simulink model "Despegue_model"  (R2015b)
settings: Solver=ode45  StartTime=0  StopTime=1000  FixedStep=0.001  RelTol=1e-3
libraries: simulink_extras x4, aerolibtransform2 x2, aerolibutil x2, simulink x1, aerolibobsolete x1, aerolibasang x1
settings Model: Creator=David  LastModifiedBy=Juan
settings SolverCC: InitialStep=AUTO
settings DataIOCC: SaveCompleteFinalSimState=on  SaveFormat=Array  SaveState=on  ReturnWorkspaceOutputsName=simout
settings DebuggingCC: AlgebraicLoopMsg=none  UnderspecifiedInitializationDetection=Classic  MergeDetectMultiDrivingBlocksExec=none  StateNameClashWarn=warning
settings HardwareCC: ProdBitPerPointer=32  ProdLargestAtomicFloat=None  ProdIntDivRoundTo=Undefined  ProdEndianess=Unspecified  ProdWordSize=32  ProdHWDeviceType=32-bit Generic
settings GRTTargetCC: GeneratePreprocessorConditionals=Disable all
settings ConfigComp: CovModelRefEnable=Off

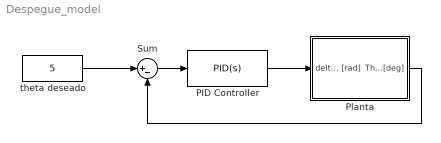
== system Despegue_model ==
  PID Controller : simulink/Continuous/PID Controller  Controller=PID  TimeDomain=Continuous-time  SampleTime=-1  IntegratorMethod=Forward Euler  FilterMethod=Forward Euler  Form=Parallel  UseFilter=on  ControllerParametersSource=internal  P=-0.450238898063441  I=-0.00789924414267895  D=0.0642858198815756  N=2  InitialConditionSource=internal  InitialConditionForIntegrator=0  InitialConditionForFilter=0  ExternalReset=none  LimitOutput=on  UpperSaturationLimit=0.062  LowerSaturationLimit=-0.062  LinearizeAsGain=on  AntiWindupMode=none  Kb=1  TrackingMode=off  Kt=1  PParamMin=[]  PParamMax=[]  IParamMin=[]  IParamMax=[]  DParamMin=[]  DParamMax=[]  NParamMin=[]  NParamMax=[]  KbParamMin=[]  KbParamMax=[]  KtParamMin=[]  KtParamMax=[]  POutMin=[]  POutMax=[]  IOutMin=[]  IOutMax=[]  DOutMin=[]  DOutMax=[]  NOutMin=[]  NOutMax=[]  KbOutMin=[]  KbOutMax=[]  KtOutMin=[]  KtOutMax=[]  IntegratorOutMin=[]  IntegratorOutMax=[]  FilterOutMin=[]  FilterOutMax=[]  SumOutMin=[]  SumOutMax=[]  SumI1OutMin=[]  SumI1OutMax=[]  SumI2OutMin=[]  SumI2OutMax=[]  SumI3OutMin=[]  SumI3OutMax=[]  SumDOutMin=[]  SumDOutMax=[]  SaturationOutMin=[]  SaturationOutMax=[]  IntegratorContinuousStateAttributes=''  IntegratorStateMustResolveToSignalObject=off  IntegratorRTWStateStorageClass=Auto  FilterContinuousStateAttributes=''  FilterStateMustResolveToSignalObject=off  FilterRTWStateStorageClass=Auto  DifferentiatorICPrevScaledInput=0  DifferentiatorOutMin=[]  DifferentiatorOutMax=[]
  Planta : Subsystem
  Sum : Sum  Inputs=|+-
  theta deseado : Constant  Value=5
  wires:
  Planta/1(Theta[deg]) -> Sum/2
  Sum/1 -> PID Controller/1
  theta deseado/1 -> Sum/1
  PID Controller/1 -> Planta/1(delta [rad])

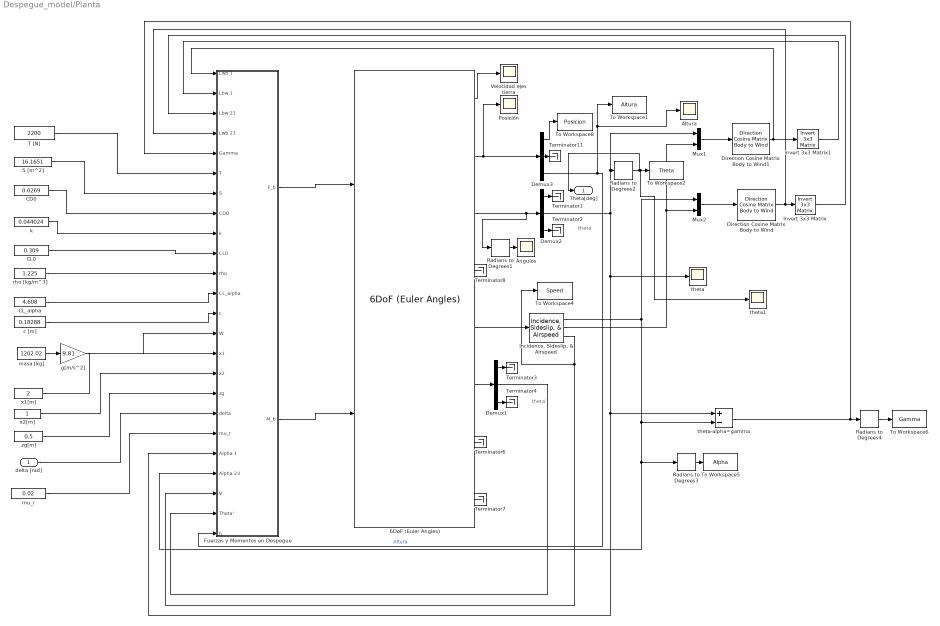
== system Despegue_model/Planta ==
  note: theta'
  note: theta
  delta [rad] : Inport
  6DoF (Euler Angles) : aerolibobsolete/6DoF (Euler Angles)  units=Metric (MKS)  mtype=Fixed  rep=Euler Angles  xme_0=[0 0 0]  Vm_0=[0.01 0 0]  eul_0=[0 0.035 0]  pm_0=[0 0 0]  mass_0=Mass  mass_e=0.5  mass_f=2.0  inertia=Inertia  inertia_e=eye(3)  inertia_f=2*eye(3)  k_quat=1.0
  Altura : Scope
  CD0 : Constant  Value=0.0269
  CL0 : Constant  Value=0.309
  "CL_alpha " : Constant  Value=4.608
  Demux1 : Demux  Outputs=3
  Demux2 : Demux  Outputs=3
  Demux3 : Demux  Outputs=3
  Direction Cosine Matrix Body to Wind : aerolibtransform2/Direction Cosine Matrix Body to Wind
  Direction Cosine Matrix Body to Wind1 : aerolibtransform2/Direction Cosine Matrix Body to Wind
  Fuerzas y Momentos en Despegue : Subsystem
  "Incidence, Sideslip, & Airspeed" : aerolibasang/Incidence, Sideslip, & Airspeed
  Invert 3x3 Matrix : aerolibutil/Invert  3x3 Matrix
  Invert 3x3 Matrix1 : aerolibutil/Invert  3x3 Matrix
  Mux1 : Mux  Inputs=2
  Mux2 : Mux  Inputs=2
  Posición : Scope
  Radians to Degrees{1..4} (4 alike) : simulink_extras/Transformations/Radians to Degrees
  S [m^2] : Constant  Value=16.1651
  T [N] : Constant  Value=2200
  Terminator{1..4,6..8,11} (8 alike) : Terminator
  To Workspace1 : ToWorkspace  VariableName=Altura  SampleTime=-1
  To Workspace2 : ToWorkspace  VariableName=Theta  SampleTime=-1
  To Workspace4 : ToWorkspace  VariableName=Speed  SampleTime=-1
  To Workspace5 : ToWorkspace  VariableName=Alpha  SampleTime=-1
  To Workspace6 : ToWorkspace  VariableName=Gamma  SampleTime=-1
  To Workspace8 : ToWorkspace  VariableName=Posicion  SampleTime=-1
  "Velocidad ejes tierra " : Scope
  c [m] : Constant  Value=0.18288
  g[m/s^2] : Gain  Gain=9.81
  k : Constant  Value=0.044024
  "masa [kg] " : Constant  Value=1202.02
  "mu_r " : Constant  Value=0.02
  rho [kg/m^3] : Constant  Value=1.225
  theta : Scope
  theta-alpha=gamma : Sum  Inputs=+-
  theta1 : Scope
  x1[m] : Constant  Value=2
  x2[m] : Constant
  zg[m] : Constant  Value=0.5
  Ángulos : Scope
  Theta[deg] : Outport
  wires:
  6DoF (Euler Angles)/1 -> "Velocidad ejes tierra "/1
  6DoF (Euler Angles)/6 -> Demux1/1
  6DoF (Euler Angles)/7 -> Terminator6/1
  6DoF (Euler Angles)/8 -> Terminator7/1
  Radians to Degrees4/1 -> To Workspace6/1
  T [N]/1 -> Fuerzas y Momentos en Despegue/6(T)
  "Incidence, Sideslip, & Airspeed"/3 -> Fuerzas y Momentos en Despegue/22(V), To Workspace4/1
  Demux2/3 -> Terminator2/1
  Invert 3x3 Matrix1/1 -> Fuerzas y Momentos en Despegue/2(Lbw 1)
  Demux1/1 -> Terminator3/1
  Demux3/2 -> Terminator11/1
  Radians to Degrees1/1 -> Ángulos/1
  S [m^2]/1 -> Fuerzas y Momentos en Despegue/7(S)
  CD0/1 -> Fuerzas y Momentos en Despegue/8(CD0)
  Demux3/1 -> To Workspace8/1
  Demux2/2 -> theta/1, Fuerzas y Momentos en Despegue/20(Alpha 1), theta-alpha=gamma/1, Mux1/1, Radians to Degrees2/1
  6DoF (Euler Angles)/2 -> Demux3/1, Posición/1
  "Incidence, Sideslip, & Airspeed"/2 -> Mux2/2, Mux1/2
  "masa [kg] "/1 -> g[m/s^2]/1
  6DoF (Euler Angles)/5 -> "Incidence, Sideslip, & Airspeed"/1
  6DoF (Euler Angles)/4 -> Terminator8/1
  Demux2/1 -> Terminator1/1
  Mux2/1 -> Direction Cosine Matrix Body to Wind/1
  Direction Cosine Matrix Body to Wind1/1 -> Fuerzas y Momentos en Despegue/1(Lwb 1), Invert 3x3 Matrix1/1
  Direction Cosine Matrix Body to Wind/1 -> Fuerzas y Momentos en Despegue/4(Lwb 23), Invert 3x3 Matrix/1
  Radians to Degrees3/1 -> To Workspace5/1
  theta-alpha=gamma/1 -> Fuerzas y Momentos en Despegue/5(Gamma), Radians to Degrees4/1
  k/1 -> Fuerzas y Momentos en Despegue/9(k)
  Invert 3x3 Matrix/1 -> Fuerzas y Momentos en Despegue/3(Lbw 23)
  Mux1/1 -> Direction Cosine Matrix Body to Wind1/1
  Demux3/3 -> Fuerzas y Momentos en Despegue/24(h), To Workspace1/1, Altura/1  "Altura"
  Radians to Degrees2/1 -> theta1/1, To Workspace2/1, Theta[deg]/1
  Demux1/3 -> Terminator4/1
  6DoF (Euler Angles)/3 -> Radians to Degrees1/1, Demux2/1
  zg[m]/1 -> Fuerzas y Momentos en Despegue/17(zg)
  CL0/1 -> Fuerzas y Momentos en Despegue/10(CL0)
  Demux1/2 -> Fuerzas y Momentos en Despegue/23(Theta')
  rho [kg/m^3]/1 -> Fuerzas y Momentos en Despegue/11(rho)
  "CL_alpha "/1 -> Fuerzas y Momentos en Despegue/12(CL_alpha)
  c [m]/1 -> Fuerzas y Momentos en Despegue/13(c)
  Fuerzas y Momentos en Despegue/1(F_b) -> 6DoF (Euler Angles)/1
  g[m/s^2]/1 -> Fuerzas y Momentos en Despegue/14(W)
  x1[m]/1 -> Fuerzas y Momentos en Despegue/15(x1)
  x2[m]/1 -> Fuerzas y Momentos en Despegue/16(x2)
  "mu_r "/1 -> Fuerzas y Momentos en Despegue/19(mu_r)
  Fuerzas y Momentos en Despegue/2(M_b) -> 6DoF (Euler Angles)/2
  delta [rad]/1 -> Fuerzas y Momentos en Despegue/18(delta)
  "Incidence, Sideslip, & Airspeed"/1 -> Mux2/1, Radians to Degrees3/1, Fuerzas y Momentos en Despegue/21(Alpha 23), theta-alpha=gamma/2

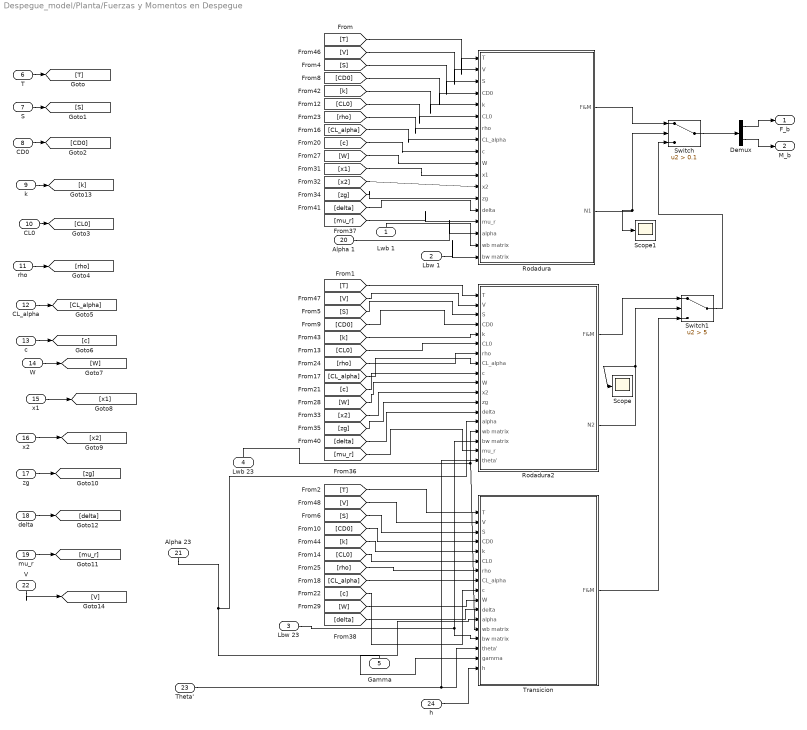
== system Despegue_model/Planta/Fuerzas y Momentos en Despegue ==
  Lwb 1 : Inport
  Lbw 1 : Inport  Port=2
  Lbw 23 : Inport  Port=3
  Lwb 23 : Inport  Port=4
  Gamma : Inport  Port=5
  T : Inport  Port=6
  S : Inport  Port=7
  CD0 : Inport  Port=8
  k : Inport  Port=9
  CL0 : Inport  Port=10
  rho : Inport  Port=11
  CL_alpha : Inport  Port=12
  c : Inport  Port=13
  W : Inport  Port=14
  x1 : Inport  Port=15
  x2 : Inport  Port=16
  zg : Inport  Port=17
  delta : Inport  Port=18
  mu_r : Inport  Port=19
  Alpha 1 : Inport  Port=20
  Alpha 23 : Inport  Port=21
  V : Inport  Port=22
  Theta' : Inport  Port=23
  h : Inport  Port=24
  Demux : Demux  Outputs=2
  Rodadura : Subsystem
  Rodadura2 : Subsystem
  Scope : Scope
  Scope1 : Scope
  Switch : Switch  Criteria=u2 > Threshold  Threshold=0.1
  Switch1 : Switch  Criteria=u2 > Threshold  Threshold=5  ZeroCross=off
  Transicion : Subsystem
  F_b : Outport
  M_b : Outport  Port=2
  wires:
  Alpha 1/1 -> Rodadura/16(alpha)
  Alpha 23/1 -> Transicion/12(alpha), Rodadura2/14(alpha)
  Gamma/1 -> Transicion/16(gamma)
  Lwb 23/1 -> Transicion/13(wb matrix), Rodadura2/15(wb matrix)
  Rodadura/1(F&M) -> Switch/1
  Theta'/1 -> Transicion/15(theta'), Rodadura2/18(theta')
  Switch1/1 -> Switch/3
  Switch/1 -> Demux/1
  Lbw 23/1 -> Transicion/14(bw matrix), Rodadura2/16(bw matrix)
  Rodadura2/1(F&M) -> Switch1/1
  Demux/2 -> M_b/1
  Lbw 1/1 -> Rodadura/18(bw matrix)
  Rodadura2/2("N2 ") -> Scope/1, Switch1/2
  Demux/1 -> F_b/1
  T/1 -> [T]
  [T] -> Rodadura/1(T)
  [T] -> Rodadura2/1(T)
  [T] -> Transicion/1(T)
  S/1 -> [S]
  CD0/1 -> [CD0]
  CL0/1 -> [CL0]
  rho/1 -> [rho]
  CL_alpha/1 -> [CL_alpha]
  c/1 -> [c]
  W/1 -> [W]
  x1/1 -> [x1]
  x2/1 -> [x2]
  zg/1 -> [zg]
  [S] -> Rodadura/3(S)
  [S] -> Rodadura2/3(S)
  [S] -> Transicion/3(S)
  [CD0] -> Rodadura/4(CD0)
  [CD0] -> Rodadura2/4(CD0)
  [CD0] -> Transicion/4(CD0)
  [CL0] -> Rodadura/6(CL0)
  [CL0] -> Rodadura2/6(CL0)
  [CL0] -> Transicion/6(CL0)
  [CL_alpha] -> Rodadura/8(CL_alpha)
  [CL_alpha] -> Rodadura2/8(CL_alpha)
  [CL_alpha] -> Transicion/8(CL_alpha)
  [c] -> Rodadura/9(c)
  [c] -> Rodadura2/9(c)
  [c] -> Transicion/9(c)
  [rho] -> Rodadura/7(rho)
  [rho] -> Rodadura2/7(rho)
  [rho] -> Transicion/7(rho)
  [W] -> Rodadura/10(W)
  [W] -> Rodadura2/10(W)
  [W] -> Transicion/10(W)
  [x1] -> Rodadura/11(x1)
  [x2] -> Rodadura/12(x2)
  [x2] -> Rodadura2/11(x2)
  [zg] -> Rodadura/13(zg)
  [zg] -> Rodadura2/12(zg)
  mu_r/1 -> [mu_r]
  [mu_r] -> Rodadura2/17(mu_r)
  [mu_r] -> Rodadura/15(mu_r)
  delta/1 -> [delta]
  [delta] -> Transicion/11(delta)
  [delta] -> Rodadura2/13(delta)
  [delta] -> Rodadura/14(delta)
  k/1 -> [k]
  [k] -> Rodadura/5(k)
  [k] -> Rodadura2/5(k)
  [k] -> Transicion/5(k)
  V/1 -> [V]
  [V] -> Rodadura/2(V)
  [V] -> Rodadura2/2(V)
  [V] -> Transicion/2(V)
  Lwb 1/1 -> Rodadura/17(wb matrix)
  Transicion/1(F&M) -> Switch1/3
  Rodadura/2("N1 ") -> Switch/2, Scope1/1
  h/1 -> Transicion/17(h)

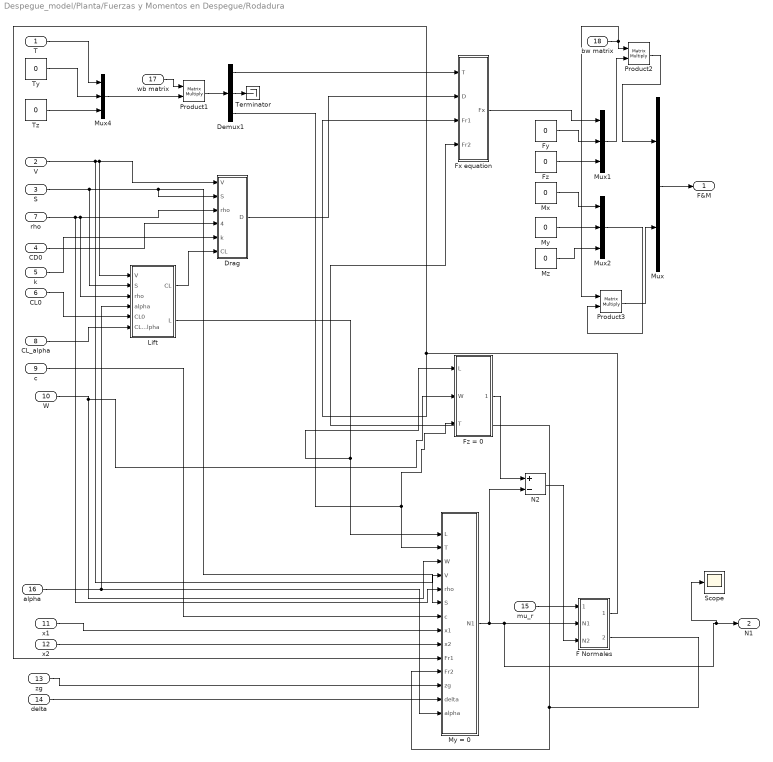
== system Despegue_model/Planta/Fuerzas y Momentos en Despegue/Rodadura ==
  T : Inport
  V : Inport  Port=2
  S : Inport  Port=3
  CD0 : Inport  Port=4
  k : Inport  Port=5
  CL0 : Inport  Port=6
  rho : Inport  Port=7
  CL_alpha : Inport  Port=8
  c : Inport  Port=9
  W : Inport  Port=10
  x1 : Inport  Port=11
  x2 : Inport  Port=12
  zg : Inport  Port=13
  delta : Inport  Port=14
  mu_r : Inport  Port=15
  alpha : Inport  Port=16
  wb matrix : Inport  Port=17
  bw matrix : Inport  Port=18
  Demux1 : Demux  Outputs=3
  Drag : Subsystem
  F Normales : Subsystem
  Fx equation : Subsystem
  Fy : Constant  Value=0
  Fz : Constant  Value=0
  Fz = 0 : Subsystem
  Lift : Subsystem
  Mux : Mux  Inputs=2
  Mux1 : Mux  Inputs=3
  Mux2 : Mux  Inputs=3
  Mux4 : Mux  Inputs=3
  Mx : Constant  Value=0
  My : Constant  Value=0
  My = 0 : Subsystem
  Mz : Constant  Value=0
  N2 : Sum  Inputs=+-
  Product1 : Product  Multiplication=Matrix(*)
  Product2 : Product  Multiplication=Matrix(*)
  Product3 : Product  Multiplication=Matrix(*)
  Scope : Scope
  Terminator : Terminator
  Ty : Constant  Value=0
  Tz : Constant  Value=0
  F&M : Outport
  "N1 " : Outport  Port=2
  wires:
  Mux/1 -> F&M/1
  Fz/1 -> Mux1/3
  Mx/1 -> Mux2/1
  Mz/1 -> Mux2/3
  T/1 -> Mux4/1
  Ty/1 -> Mux4/2
  Tz/1 -> Mux4/3
  Mux4/1 -> Product1/2
  Lift/1(CL) -> Drag/6(CL)
  Lift/2(L) -> My = 0/1(L), Fz = 0/1(L)
  Drag/1(D) -> Fx equation/2(D)
  My = 0/1(N1) -> N2/2, Scope/1, "N1 "/1, F Normales/2(N1)
  Fz = 0/1(N1+N2) -> N2/1
  N2/1 -> F Normales/3(N2)
  F Normales/1("Fr1 ") -> Fx equation/3(Fr1), My = 0/10(Fr1)
  F Normales/2(Fr2) -> My = 0/11(Fr2), Fx equation/4(Fr2)
  Product1/1 -> Demux1/1
  Demux1/1 -> Fx equation/1(T)
  Demux1/2 -> Terminator/1
  Demux1/3 -> My = 0/2(T), Fz = 0/3(T)
  My/1 -> Mux2/2
  Fy/1 -> Mux1/2
  V/1 -> My = 0/4(V), Lift/1(V), Drag/1(V)
  S/1 -> My = 0/6(S), Drag/2(S), Lift/2(S)
  rho/1 -> Lift/3(rho), Drag/3(rho), My = 0/5(rho)
  CD0/1 -> Drag/4(CD0)
  k/1 -> Drag/5(k)
  CL0/1 -> Lift/5(CL0)
  CL_alpha/1 -> Lift/6(CL_alpha)
  c/1 -> My = 0/7(c)
  W/1 -> My = 0/3(W), Fz = 0/2(W)
  x1/1 -> My = 0/8(x1)
  x2/1 -> My = 0/9(x2)
  zg/1 -> My = 0/12(zg)
  delta/1 -> My = 0/13(delta)
  alpha/1 -> Lift/4(alpha), My = 0/14(alpha)
  mu_r/1 -> F Normales/1(mu_r)
  wb matrix/1 -> Product1/1
  Mux1/1 -> Product2/2
  bw matrix/1 -> Product2/1, Product3/1
  Product2/1 -> Mux/1
  Product3/1 -> Mux/2
  Mux2/1 -> Product3/2
  Fx equation/1(Fx) -> Mux1/1

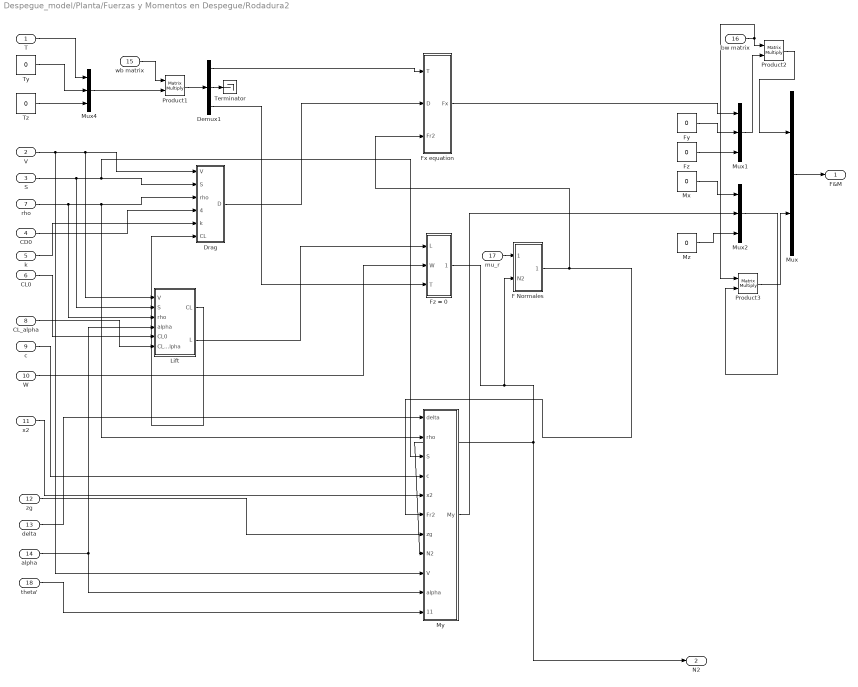
== system Despegue_model/Planta/Fuerzas y Momentos en Despegue/Rodadura2 ==
  T : Inport
  V : Inport  Port=2
  S : Inport  Port=3
  CD0 : Inport  Port=4
  k : Inport  Port=5
  CL0 : Inport  Port=6
  rho : Inport  Port=7
  CL_alpha : Inport  Port=8
  c : Inport  Port=9
  W : Inport  Port=10
  x2 : Inport  Port=11
  zg : Inport  Port=12
  delta : Inport  Port=13
  alpha : Inport  Port=14
  wb matrix : Inport  Port=15
  bw matrix : Inport  Port=16
  mu_r : Inport  Port=17
  theta' : Inport  Port=18
  " My" : Subsystem
  Demux1 : Demux  Outputs=3
  Drag : Subsystem
  F Normales : Subsystem
  Fx equation : Subsystem
  Fy : Constant  Value=0
  Fz : Constant  Value=0
  Fz = 0 : Subsystem
  Lift : Subsystem
  Mux : Mux  Inputs=2
  Mux1 : Mux  Inputs=3
  Mux2 : Mux  Inputs=3
  Mux4 : Mux  Inputs=3
  Mx : Constant  Value=0
  Mz : Constant  Value=0
  Product1 : Product  Multiplication=Matrix(*)
  Product2 : Product  Multiplication=Matrix(*)
  Product3 : Product  Multiplication=Matrix(*)
  Terminator : Terminator
  Ty : Constant  Value=0
  Tz : Constant  Value=0
  F&M : Outport
  "N2 " : Outport  Port=2
  wires:
  Mux/1 -> F&M/1
  Fz/1 -> Mux1/3
  Mx/1 -> Mux2/1
  Mz/1 -> Mux2/3
  T/1 -> Mux4/1
  Ty/1 -> Mux4/2
  Tz/1 -> Mux4/3
  Mux4/1 -> Product1/2
  Lift/1(CL) -> Drag/6(CL)
  Drag/1(D) -> Fx equation/2(D)
  Product1/1 -> Demux1/1
  Demux1/1 -> Fx equation/1(T)
  Demux1/2 -> Terminator/1
  " My"/1(My) -> Mux2/2
  Fy/1 -> Mux1/2
  V/1 -> " My"/9(V), Lift/1(V), Drag/1(V)
  S/1 -> " My"/3(S), Drag/2(S), Lift/2(S)
  rho/1 -> Lift/3(rho), " My"/2(rho), Drag/3(rho)
  CD0/1 -> Drag/4(CD0)
  k/1 -> Drag/5(k)
  CL0/1 -> Lift/5(CL0)
  CL_alpha/1 -> Lift/6(CL_alpha)
  W/1 -> Fz = 0/2(W)
  alpha/1 -> Lift/4(alpha), " My"/10(alpha)
  wb matrix/1 -> Product1/1
  Mux1/1 -> Product2/2
  bw matrix/1 -> Product2/1, Product3/1
  Product2/1 -> Mux/1
  Product3/1 -> Mux/2
  Mux2/1 -> Product3/2
  Fz = 0/1(N2) -> "N2 "/1, " My"/8(N2), F Normales/2(N2)
  mu_r/1 -> F Normales/1(mu_r)
  F Normales/1(Fr2) -> Fx equation/3(Fr2), " My"/6(Fr2)
  Lift/2(L) -> Fz = 0/1(L)
  Demux1/3 -> Fz = 0/3(T)
  delta/1 -> " My"/1(delta)
  c/1 -> " My"/4(c)
  zg/1 -> " My"/7(zg)
  x2/1 -> " My"/5(x2)
  theta'/1 -> " My"/11(theta')
  Fx equation/1(Fx) -> Mux1/1

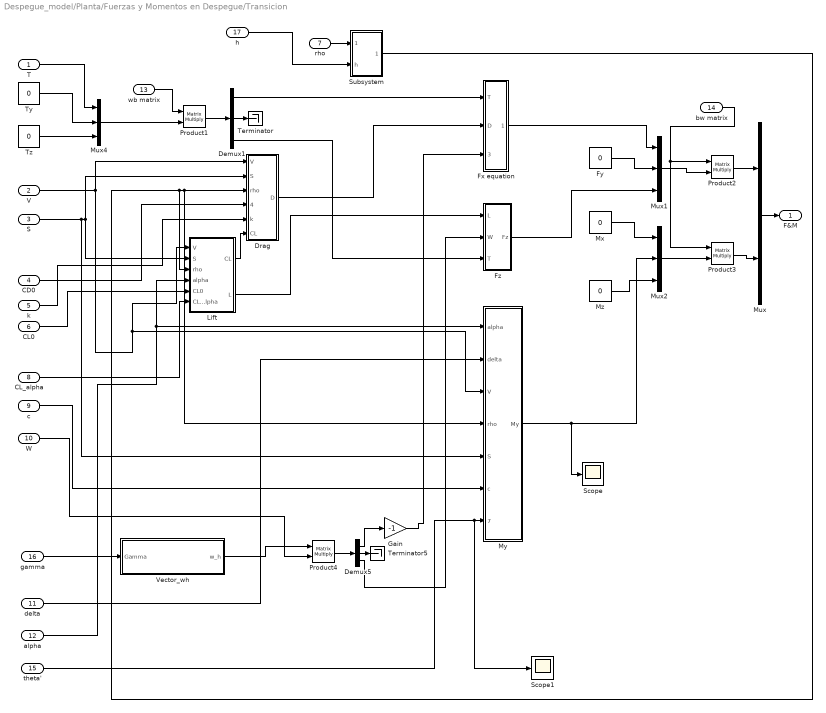
== system Despegue_model/Planta/Fuerzas y Momentos en Despegue/Transicion ==
  T : Inport
  V : Inport  Port=2
  S : Inport  Port=3
  CD0 : Inport  Port=4
  k : Inport  Port=5
  CL0 : Inport  Port=6
  rho : Inport  Port=7
  CL_alpha : Inport  Port=8
  c : Inport  Port=9
  W : Inport  Port=10
  delta : Inport  Port=11
  alpha : Inport  Port=12
  wb matrix : Inport  Port=13
  bw matrix : Inport  Port=14
  theta' : Inport  Port=15
  gamma : Inport  Port=16
  h : Inport  Port=17
  " My" : Subsystem
  Demux1 : Demux  Outputs=3
  Demux5 : Demux  Outputs=3
  Drag : Subsystem
  Fx equation : Subsystem
  Fy : Constant  Value=0
  "Fz " : Subsystem
  Gain : Gain  Gain=-1
  Lift : Subsystem
  Mux : Mux  Inputs=2
  Mux1 : Mux  Inputs=3
  Mux2 : Mux  Inputs=3
  Mux4 : Mux  Inputs=3
  Mx : Constant  Value=0
  Mz : Constant  Value=0
  Product{1..4} (4 alike) : Product  Multiplication=Matrix(*)
  Scope : Scope
  Scope1 : Scope
  Subsystem : Subsystem
  Terminator : Terminator
  Terminator5 : Terminator
  Ty : Constant  Value=0
  Tz : Constant  Value=0
  Vector_wh : Subsystem
  F&M : Outport
  wires:
  Mux/1 -> F&M/1
  Mx/1 -> Mux2/1
  Mz/1 -> Mux2/3
  T/1 -> Mux4/1
  Ty/1 -> Mux4/2
  Tz/1 -> Mux4/3
  Mux4/1 -> Product1/2
  Lift/1(CL) -> Drag/6(CL)
  Product1/1 -> Demux1/1
  Demux1/1 -> Fx equation/1(T)
  Demux1/2 -> Terminator/1
  Fy/1 -> Mux1/2
  V/1 -> " My"/3(V), Lift/1(V), Drag/1(V)
  S/1 -> " My"/5(S), Drag/2(S), Lift/2(S)
  CD0/1 -> Drag/4(CD0)
  k/1 -> Drag/5(k)
  CL0/1 -> Lift/5(CL0)
  CL_alpha/1 -> Lift/6(CL_alpha)
  alpha/1 -> " My"/1(alpha), Lift/4(alpha)
  wb matrix/1 -> Product1/1
  Mux1/1 -> Product2/2
  bw matrix/1 -> Product3/1, Product2/1
  Product2/1 -> Mux/1
  Product3/1 -> Mux/2
  Mux2/1 -> Product3/2
  gamma/1 -> Vector_wh/1(Gamma)
  Demux5/2 -> Terminator5/1
  Product4/1 -> Demux5/1
  W/1 -> Product4/2
  Vector_wh/1(w_h) -> Product4/1
  Demux5/1 -> Gain/1
  Gain/1 -> Fx equation/3(W)
  Demux5/3 -> "Fz "/2(W)
  Drag/1(D) -> Fx equation/2(D)
  c/1 -> " My"/6(c)
  delta/1 -> " My"/2(delta)
  Demux1/3 -> "Fz "/3(T)
  " My"/1(My) -> Scope/1, Mux2/2
  "Fz "/1(Fz) -> Mux1/3
  theta'/1 -> Scope1/1, " My"/7(theta')
  Fx equation/1(Fx) -> Mux1/1
  Lift/2(L) -> "Fz "/1(L)
  rho/1 -> Subsystem/1(rho)
  h/1 -> Subsystem/2(h)
  Subsystem/1(Out1) -> " My"/4(rho), Drag/3(rho), Lift/3(rho)

== system Despegue_model/Planta/Fuerzas y Momentos en Despegue/Rodadura/Drag ==
  V : Inport
  S : Inport  Port=2
  rho : Inport  Port=3
  CD0 : Inport  Port=4
  k : Inport  Port=5
  CL : Inport  Port=6
  CD : Subsystem
  Drag : Subsystem
  D : Outport
  wires:
  V/1 -> Drag/1(V)
  rho/1 -> Drag/3(rho)
  S/1 -> Drag/2(S)
  Drag/1(D) -> D/1
  CD/1(CD) -> Drag/4(CD)
  CL/1 -> CD/3(CL)
  CD0/1 -> CD/1(CD0)
  k/1 -> CD/2(k)

== system Despegue_model/Planta/Fuerzas y Momentos en Despegue/Rodadura/F Normales ==
  mu_r : Inport
  N1 : Inport  Port=2
  N2 : Inport  Port=3
  Product : Product
  Product1 : Product
  "Fr1 " : Outport
  Fr2 : Outport  Port=2
  wires:
  mu_r/1 -> Product/1, Product1/1
  N1/1 -> Product/2
  N2/1 -> Product1/2
  Product/1 -> "Fr1 "/1
  Product1/1 -> Fr2/1

== system Despegue_model/Planta/Fuerzas y Momentos en Despegue/Rodadura/Fx equation ==
  T : Inport
  D : Inport  Port=2
  Fr1 : Inport  Port=3
  Fr2 : Inport  Port=4
  Add : Sum
  Add2 : Sum  Inputs=+++
  Gain : Gain  Gain=-1
  Gain2 : Gain  Gain=-1
  Fx : Outport
  wires:
  Add/1 -> Gain2/1
  Fr1/1 -> Add/1
  Add2/1 -> Fx/1
  Gain/1 -> Add2/2
  Fr2/1 -> Add/2
  D/1 -> Gain/1
  Gain2/1 -> Add2/3
  T/1 -> Add2/1

== system Despegue_model/Planta/Fuerzas y Momentos en Despegue/Rodadura/Fz = 0 ==
  L : Inport
  W : Inport  Port=2
  T : Inport  Port=3
  Add1 : Sum  Inputs=+--
  N1+N2 : Outport
  wires:
  L/1 -> Add1/2
  Add1/1 -> N1+N2/1
  W/1 -> Add1/1
  T/1 -> Add1/3

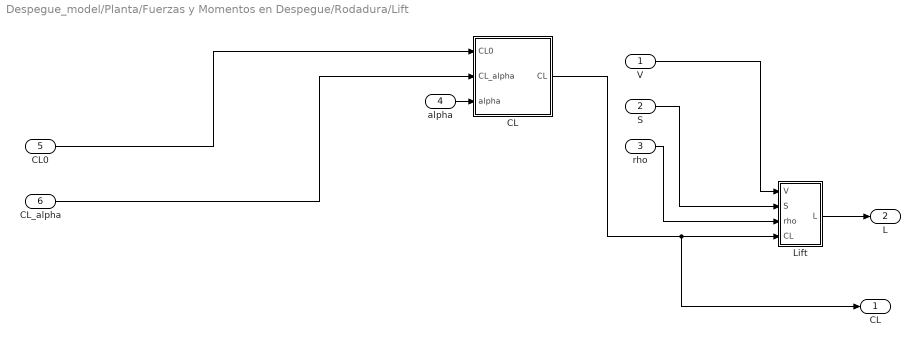
== system Despegue_model/Planta/Fuerzas y Momentos en Despegue/Rodadura/Lift ==
  V : Inport
  S : Inport  Port=2
  rho : Inport  Port=3
  alpha : Inport  Port=4
  CL0 : Inport  Port=5
  CL_alpha : Inport  Port=6
  "CL " : Subsystem
  Lift : Subsystem
  CL : Outport
  L : Outport  Port=2
  wires:
  rho/1 -> Lift/3(rho)
  S/1 -> Lift/2(S)
  V/1 -> Lift/1(V)
  "CL "/1("CL ") -> CL/1, Lift/4(CL)
  CL0/1 -> "CL "/1(CL0)
  CL_alpha/1 -> "CL "/2(CL_alpha)
  alpha/1 -> "CL "/3(alpha)
  Lift/1(L) -> L/1

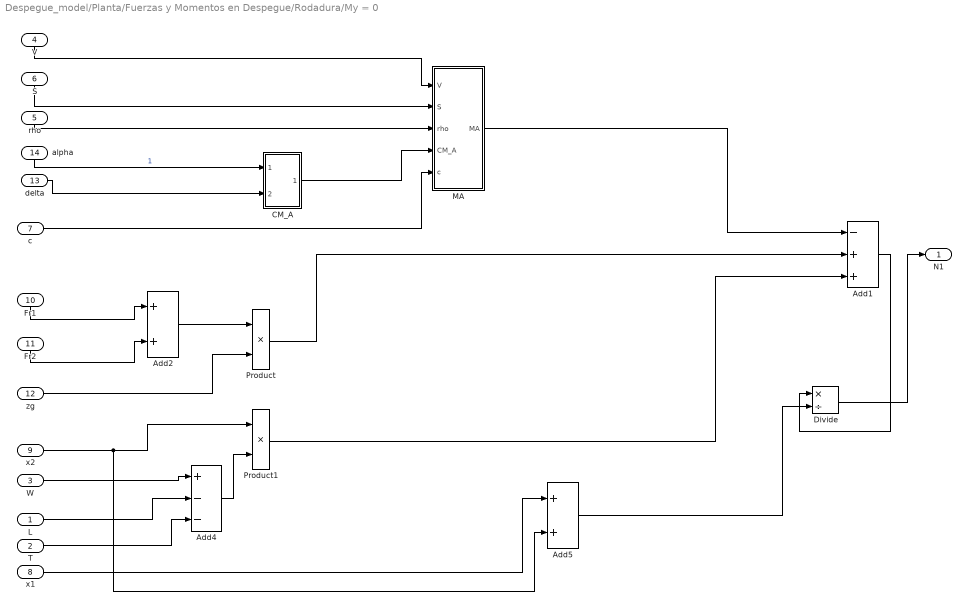
== system Despegue_model/Planta/Fuerzas y Momentos en Despegue/Rodadura/My = 0 ==
  L : Inport
  T : Inport  Port=2
  W : Inport  Port=3
  V : Inport  Port=4
  rho : Inport  Port=5
  S : Inport  Port=6
  c : Inport  Port=7
  x1 : Inport  Port=8
  x2 : Inport  Port=9
  Fr1 : Inport  Port=10
  Fr2 : Inport  Port=11
  zg : Inport  Port=12
  delta : Inport  Port=13
  alpha : Inport  Port=14
  Add1 : Sum  Inputs=-++
  Add2 : Sum
  Add4 : Sum  Inputs=+--
  Add5 : Sum
  CM_A : Subsystem
  Divide : Product  Inputs=*/
  MA : Subsystem
  Product : Product
  Product1 : Product
  N1 : Outport
  wires:
  alpha/1 -> CM_A/1(alpha)  "1"
  CM_A/1(CM_A) -> MA/4(CM_A)
  delta/1 -> CM_A/2(delta)
  c/1 -> MA/5(c)
  MA/1(MA) -> Add1/1
  Fr1/1 -> Add2/1
  Fr2/1 -> Add2/2
  Add2/1 -> Product/1
  zg/1 -> Product/2
  x2/1 -> Add5/2, Product1/1
  Add4/1 -> Product1/2
  Product/1 -> Add1/2
  Product1/1 -> Add1/3
  x1/1 -> Add5/1
  Add1/1 -> Divide/1
  Add5/1 -> Divide/2
  Divide/1 -> N1/1
  W/1 -> Add4/1
  L/1 -> Add4/2
  V/1 -> MA/1(V)
  S/1 -> MA/2(S)
  rho/1 -> MA/3(rho)
  T/1 -> Add4/3

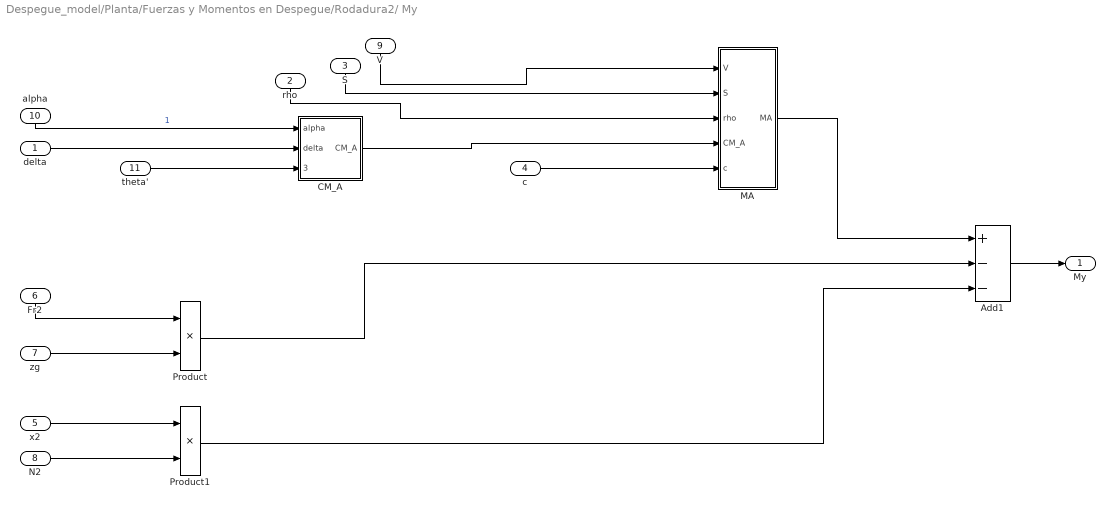
== system Despegue_model/Planta/Fuerzas y Momentos en Despegue/Rodadura2/ My ==
  delta : Inport
  rho : Inport  Port=2
  S : Inport  Port=3
  c : Inport  Port=4
  x2 : Inport  Port=5
  Fr2 : Inport  Port=6
  zg : Inport  Port=7
  N2 : Inport  Port=8
  V : Inport  Port=9
  alpha : Inport  Port=10
  theta' : Inport  Port=11
  Add1 : Sum  Inputs=+--
  CM_A : Subsystem
  MA : Subsystem
  Product : Product
  Product1 : Product
  My : Outport
  wires:
  alpha/1 -> CM_A/1(alpha)  "1"
  V/1 -> MA/1(V)
  rho/1 -> MA/3(rho)
  S/1 -> MA/2(S)
  CM_A/1(CM_A) -> MA/4(CM_A)
  delta/1 -> CM_A/2(delta)
  c/1 -> MA/5(c)
  MA/1(MA) -> Add1/1
  Fr2/1 -> Product/1
  zg/1 -> Product/2
  x2/1 -> Product1/1
  Product/1 -> Add1/2
  Product1/1 -> Add1/3
  Add1/1 -> My/1
  N2/1 -> Product1/2
  theta'/1 -> CM_A/3(theta')

== system Despegue_model/Planta/Fuerzas y Momentos en Despegue/Rodadura2/Drag ==
  V : Inport
  S : Inport  Port=2
  rho : Inport  Port=3
  CD0 : Inport  Port=4
  k : Inport  Port=5
  CL : Inport  Port=6
  CD : Subsystem
  Drag : Subsystem
  D : Outport
  wires:
  V/1 -> Drag/1(V)
  rho/1 -> Drag/3(rho)
  S/1 -> Drag/2(S)
  Drag/1(D) -> D/1
  CD/1(CD) -> Drag/4(CD)
  CL/1 -> CD/3(CL)
  CD0/1 -> CD/1(CD0)
  k/1 -> CD/2(k)

== system Despegue_model/Planta/Fuerzas y Momentos en Despegue/Rodadura2/F Normales ==
  mu_r : Inport
  N2 : Inport  Port=2
  Product1 : Product
  Fr2 : Outport
  wires:
  mu_r/1 -> Product1/1
  N2/1 -> Product1/2
  Product1/1 -> Fr2/1

== system Despegue_model/Planta/Fuerzas y Momentos en Despegue/Rodadura2/Fx equation ==
  T : Inport
  D : Inport  Port=2
  Fr2 : Inport  Port=3
  Add2 : Sum  Inputs=+++
  Gain : Gain  Gain=-1
  Gain2 : Gain  Gain=-1
  Fx : Outport
  wires:
  Fr2/1 -> Gain2/1
  Add2/1 -> Fx/1
  Gain/1 -> Add2/2
  D/1 -> Gain/1
  Gain2/1 -> Add2/3
  T/1 -> Add2/1

== system Despegue_model/Planta/Fuerzas y Momentos en Despegue/Rodadura2/Fz = 0 ==
  L : Inport
  W : Inport  Port=2
  T : Inport  Port=3
  Add1 : Sum  Inputs=+--
  Scope : Scope
  N2 : Outport
  wires:
  Add1/1 -> N2/1
  L/1 -> Scope/1, Add1/2
  W/1 -> Add1/1
  T/1 -> Add1/3

== system Despegue_model/Planta/Fuerzas y Momentos en Despegue/Rodadura2/Lift ==
  V : Inport
  S : Inport  Port=2
  rho : Inport  Port=3
  alpha : Inport  Port=4
  CL0 : Inport  Port=5
  CL_alpha : Inport  Port=6
  "CL " : Subsystem
  Lift : Subsystem
  CL : Outport
  L : Outport  Port=2
  wires:
  rho/1 -> Lift/3(rho)
  S/1 -> Lift/2(S)
  V/1 -> Lift/1(V)
  "CL "/1("CL ") -> CL/1, Lift/4(CL)
  CL0/1 -> "CL "/1(CL0)
  CL_alpha/1 -> "CL "/2(CL_alpha)
  alpha/1 -> "CL "/3(alpha)
  Lift/1(L) -> L/1

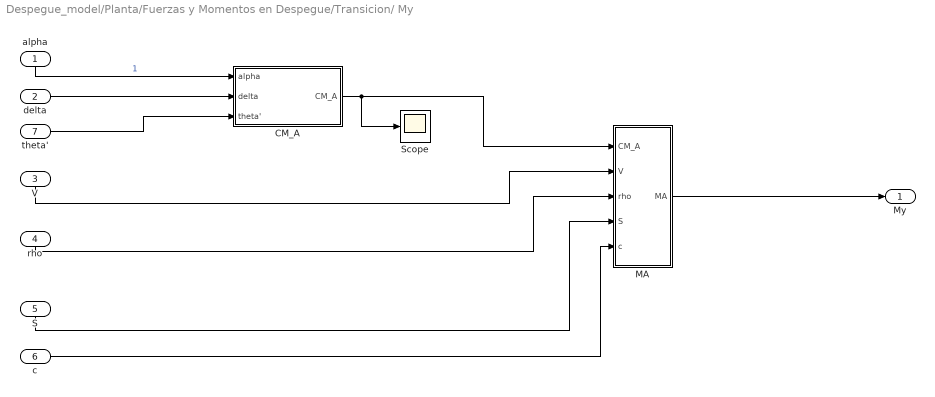
== system Despegue_model/Planta/Fuerzas y Momentos en Despegue/Transicion/ My ==
  alpha : Inport
  delta : Inport  Port=2
  V : Inport  Port=3
  rho : Inport  Port=4
  S : Inport  Port=5
  c : Inport  Port=6
  theta' : Inport  Port=7
  CM_A : Subsystem
  MA : Subsystem
  Scope : Scope
  My : Outport
  wires:
  alpha/1 -> CM_A/1(alpha)  "1"
  V/1 -> MA/2(V)
  rho/1 -> MA/3(rho)
  S/1 -> MA/4(S)
  delta/1 -> CM_A/2(delta)
  c/1 -> MA/5(c)
  theta'/1 -> CM_A/3(theta')
  MA/1(MA) -> My/1
  CM_A/1(CM_A) -> Scope/1, MA/1(CM_A)

== system Despegue_model/Planta/Fuerzas y Momentos en Despegue/Transicion/Drag ==
  V : Inport
  S : Inport  Port=2
  rho : Inport  Port=3
  CD0 : Inport  Port=4
  k : Inport  Port=5
  CL : Inport  Port=6
  CD : Subsystem
  Drag : Subsystem
  D : Outport
  wires:
  V/1 -> Drag/1(V)
  rho/1 -> Drag/3(rho)
  S/1 -> Drag/2(S)
  Drag/1(D) -> D/1
  CD/1(CD) -> Drag/4(CD)
  CL/1 -> CD/3(CL)
  CD0/1 -> CD/1(CD0)
  k/1 -> CD/2(k)

== system Despegue_model/Planta/Fuerzas y Momentos en Despegue/Transicion/Fx equation ==
  T : Inport
  D : Inport  Port=2
  W : Inport  Port=3
  Add2 : Sum  Inputs=+++
  Gain : Gain  Gain=-1
  Fx : Outport
  wires:
  Add2/1 -> Fx/1
  T/1 -> Add2/1
  Gain/1 -> Add2/2
  D/1 -> Gain/1
  W/1 -> Add2/3

== system Despegue_model/Planta/Fuerzas y Momentos en Despegue/Transicion/Fz  ==
  L : Inport
  W : Inport  Port=2
  T : Inport  Port=3
  Add1 : Sum  Inputs=+-+
  Scope1 : Scope
  Scope2 : Scope
  Fz : Outport
  wires:
  Add1/1 -> Fz/1
  L/1 -> Add1/2
  T/1 -> Scope1/1, Add1/3
  W/1 -> Scope2/1, Add1/1

== system Despegue_model/Planta/Fuerzas y Momentos en Despegue/Transicion/Lift ==
  V : Inport
  S : Inport  Port=2
  rho : Inport  Port=3
  alpha : Inport  Port=4
  CL0 : Inport  Port=5
  CL_alpha : Inport  Port=6
  "CL " : Subsystem
  Lift : Subsystem
  CL : Outport
  L : Outport  Port=2
  wires:
  rho/1 -> Lift/3(rho)
  S/1 -> Lift/2(S)
  V/1 -> Lift/1(V)
  "CL "/1("CL ") -> CL/1, Lift/4(CL)
  CL0/1 -> "CL "/1(CL0)
  CL_alpha/1 -> "CL "/2(CL_alpha)
  alpha/1 -> "CL "/3(alpha)
  Lift/1(L) -> L/1

== system Despegue_model/Planta/Fuerzas y Momentos en Despegue/Transicion/Subsystem ==
  rho : Inport
  h : Inport  Port=2
  Add : Sum
  Constant : Constant  Value=0.000022558
  Constant1 : Constant
  Constant2 : Constant  Value=4.2559
  Math Function : Math  Operator=pow  SaturateOnIntegerOverflow=on
  Product : Product
  Product5 : Product
  Out1 : Outport
  wires:
  Constant2/1 -> Math Function/2
  Math Function/1 -> Product5/1
  Add/1 -> Math Function/1
  rho/1 -> Product5/2
  Constant/1 -> Product/2
  Product5/1 -> Out1/1
  Product/1 -> Add/1
  Constant1/1 -> Add/2
  h/1 -> Product/1

== system Despegue_model/Planta/Fuerzas y Momentos en Despegue/Transicion/Vector_wh ==
  Gamma : Inport
  Mux : Mux  Inputs=3
  Trigonometric Function : Trigonometry
  Trigonometric Function1 : Trigonometry  Operator=cos
  Trigonometric Function2 : Trigonometry  Operator=cos
  w_h : Outport
  wires:
  Gamma/1 -> Trigonometric Function2/1, Trigonometric Function1/1, Trigonometric Function/1
  Trigonometric Function/1 -> Mux/1
  Trigonometric Function1/1 -> Mux/2
  Trigonometric Function2/1 -> Mux/3
  Mux/1 -> w_h/1

== system Despegue_model/Planta/Fuerzas y Momentos en Despegue/Rodadura/Drag/CD ==
  CD0 : Inport
  k : Inport  Port=2
  CL : Inport  Port=3
  Add : Sum
  Product : Product  Inputs=3
  CD : Outport
  wires:
  CD0/1 -> Add/1
  Product/1 -> Add/2
  k/1 -> Product/1
  Add/1 -> CD/1
  CL/1 -> Product/3, Product/2

== system Despegue_model/Planta/Fuerzas y Momentos en Despegue/Rodadura/Drag/Drag ==
  V : Inport
  S : Inport  Port=2
  rho : Inport  Port=3
  CD : Inport  Port=4
  "0.5 " : Constant  Value=0.5
  Product : Product  Inputs=6
  D : Outport
  wires:
  rho/1 -> Product/2
  V/1 -> Product/4, Product/5
  CD/1 -> Product/6
  Product/1 -> D/1
  S/1 -> Product/3
  "0.5 "/1 -> Product/1

== system Despegue_model/Planta/Fuerzas y Momentos en Despegue/Rodadura/Lift/CL  ==
  CL0 : Inport
  CL_alpha : Inport  Port=2
  alpha : Inport  Port=3
  Add : Sum
  Product : Product
  "CL " : Outport
  wires:
  CL0/1 -> Add/1
  CL_alpha/1 -> Product/1
  Product/1 -> Add/2
  alpha/1 -> Product/2
  Add/1 -> "CL "/1

== system Despegue_model/Planta/Fuerzas y Momentos en Despegue/Rodadura/Lift/Lift ==
  V : Inport
  S : Inport  Port=2
  rho : Inport  Port=3
  CL : Inport  Port=4
  "0.5 " : Constant  Value=0.5
  Product : Product  Inputs=6
  L : Outport
  wires:
  rho/1 -> Product/2
  V/1 -> Product/4, Product/5
  CL/1 -> Product/6
  Product/1 -> L/1
  S/1 -> Product/3
  "0.5 "/1 -> Product/1

== system Despegue_model/Planta/Fuerzas y Momentos en Despegue/Rodadura/My = 0/CM_A ==
  alpha : Inport
  delta : Inport  Port=2
  Add : Sum  Inputs=+++
  Cm0 : Constant  Value=0.04
  Cm_alpha : Constant  Value=-0.65
  Cm_delta : Constant  Value=-1.369
  Product : Product
  Product1 : Product
  CM_A : Outport
  wires:
  Product/1 -> Add/2
  Product1/1 -> Add/3
  Add/1 -> CM_A/1
  Cm_delta/1 -> Product1/1
  delta/1 -> Product1/2
  Cm0/1 -> Add/1
  Cm_alpha/1 -> Product/2
  alpha/1 -> Product/1

== system Despegue_model/Planta/Fuerzas y Momentos en Despegue/Rodadura/My = 0/MA ==
  V : Inport
  S : Inport  Port=2
  rho : Inport  Port=3
  CM_A : Inport  Port=4
  c : Inport  Port=5
  "0.5 " : Constant  Value=0.5
  Product : Product  Inputs=7
  MA : Outport
  wires:
  rho/1 -> Product/2
  V/1 -> Product/4, Product/5
  CM_A/1 -> Product/7
  Product/1 -> MA/1
  S/1 -> Product/3
  "0.5 "/1 -> Product/1
  c/1 -> Product/6

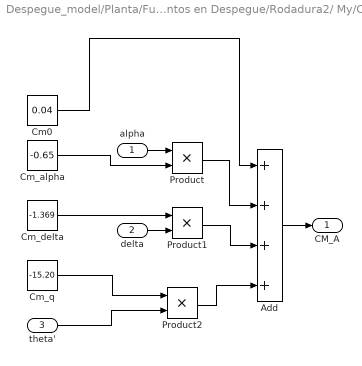
== system Despegue_model/Planta/Fuerzas y Momentos en Despegue/Rodadura2/ My/CM_A ==
  alpha : Inport
  delta : Inport  Port=2
  theta' : Inport  Port=3
  Add : Sum  Inputs=++++
  Cm0 : Constant  Value=0.04
  Cm_alpha : Constant  Value=-0.65
  Cm_delta : Constant  Value=-1.369
  Cm_q : Constant  Value=-15.20
  Product : Product
  Product1 : Product
  Product2 : Product
  CM_A : Outport
  wires:
  Product/1 -> Add/2
  Product1/1 -> Add/3
  Add/1 -> CM_A/1
  Cm_delta/1 -> Product1/1
  delta/1 -> Product1/2
  Cm0/1 -> Add/1
  Cm_alpha/1 -> Product/2
  alpha/1 -> Product/1
  Cm_q/1 -> Product2/1
  theta'/1 -> Product2/2
  Product2/1 -> Add/4

== system Despegue_model/Planta/Fuerzas y Momentos en Despegue/Rodadura2/ My/MA ==
  V : Inport
  S : Inport  Port=2
  rho : Inport  Port=3
  CM_A : Inport  Port=4
  c : Inport  Port=5
  "0.5 " : Constant  Value=0.5
  Product : Product  Inputs=7
  MA : Outport
  wires:
  rho/1 -> Product/2
  V/1 -> Product/4, Product/5
  CM_A/1 -> Product/7
  Product/1 -> MA/1
  S/1 -> Product/3
  "0.5 "/1 -> Product/1
  c/1 -> Product/6

== system Despegue_model/Planta/Fuerzas y Momentos en Despegue/Rodadura2/Drag/CD ==
  CD0 : Inport
  k : Inport  Port=2
  CL : Inport  Port=3
  Add : Sum
  Product : Product  Inputs=3
  CD : Outport
  wires:
  CD0/1 -> Add/1
  Product/1 -> Add/2
  k/1 -> Product/1
  Add/1 -> CD/1
  CL/1 -> Product/3, Product/2

== system Despegue_model/Planta/Fuerzas y Momentos en Despegue/Rodadura2/Drag/Drag ==
  V : Inport
  S : Inport  Port=2
  rho : Inport  Port=3
  CD : Inport  Port=4
  "0.5 " : Constant  Value=0.5
  Product : Product  Inputs=6
  D : Outport
  wires:
  rho/1 -> Product/2
  V/1 -> Product/4, Product/5
  CD/1 -> Product/6
  Product/1 -> D/1
  S/1 -> Product/3
  "0.5 "/1 -> Product/1

== system Despegue_model/Planta/Fuerzas y Momentos en Despegue/Rodadura2/Lift/CL  ==
  CL0 : Inport
  CL_alpha : Inport  Port=2
  alpha : Inport  Port=3
  Add : Sum
  Product : Product
  "CL " : Outport
  wires:
  CL0/1 -> Add/1
  CL_alpha/1 -> Product/1
  Product/1 -> Add/2
  alpha/1 -> Product/2
  Add/1 -> "CL "/1

== system Despegue_model/Planta/Fuerzas y Momentos en Despegue/Rodadura2/Lift/Lift ==
  V : Inport
  S : Inport  Port=2
  rho : Inport  Port=3
  CL : Inport  Port=4
  "0.5 " : Constant  Value=0.5
  Product : Product  Inputs=6
  L : Outport
  wires:
  rho/1 -> Product/2
  V/1 -> Product/4, Product/5
  CL/1 -> Product/6
  Product/1 -> L/1
  S/1 -> Product/3
  "0.5 "/1 -> Product/1

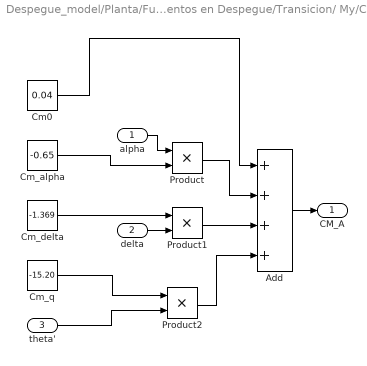
== system Despegue_model/Planta/Fuerzas y Momentos en Despegue/Transicion/ My/CM_A ==
  alpha : Inport
  delta : Inport  Port=2
  theta' : Inport  Port=3
  Add : Sum  Inputs=++++
  Cm0 : Constant  Value=0.04
  Cm_alpha : Constant  Value=-0.65
  Cm_delta : Constant  Value=-1.369
  Cm_q : Constant  Value=-15.20
  Product : Product
  Product1 : Product
  Product2 : Product
  CM_A : Outport
  wires:
  Product/1 -> Add/2
  Product1/1 -> Add/3
  Add/1 -> CM_A/1
  Cm_delta/1 -> Product1/1
  delta/1 -> Product1/2
  Cm0/1 -> Add/1
  Cm_alpha/1 -> Product/2
  alpha/1 -> Product/1
  Cm_q/1 -> Product2/1
  theta'/1 -> Product2/2
  Product2/1 -> Add/4

== system Despegue_model/Planta/Fuerzas y Momentos en Despegue/Transicion/ My/MA ==
  CM_A : Inport
  V : Inport  Port=2
  rho : Inport  Port=3
  S : Inport  Port=4
  c : Inport  Port=5
  "0.5 " : Constant  Value=0.5
  Product : Product  Inputs=7
  MA : Outport
  wires:
  rho/1 -> Product/2
  V/1 -> Product/4, Product/5
  CM_A/1 -> Product/7
  Product/1 -> MA/1
  S/1 -> Product/3
  "0.5 "/1 -> Product/1
  c/1 -> Product/6

== system Despegue_model/Planta/Fuerzas y Momentos en Despegue/Transicion/Drag/CD ==
  CD0 : Inport
  k : Inport  Port=2
  CL : Inport  Port=3
  Add : Sum
  Product : Product  Inputs=3
  CD : Outport
  wires:
  CD0/1 -> Add/1
  Product/1 -> Add/2
  k/1 -> Product/1
  Add/1 -> CD/1
  CL/1 -> Product/3, Product/2

== system Despegue_model/Planta/Fuerzas y Momentos en Despegue/Transicion/Drag/Drag ==
  V : Inport
  S : Inport  Port=2
  rho : Inport  Port=3
  CD : Inport  Port=4
  "0.5 " : Constant  Value=0.5
  Product : Product  Inputs=6
  D : Outport
  wires:
  rho/1 -> Product/2
  V/1 -> Product/4, Product/5
  CD/1 -> Product/6
  Product/1 -> D/1
  S/1 -> Product/3
  "0.5 "/1 -> Product/1

== system Despegue_model/Planta/Fuerzas y Momentos en Despegue/Transicion/Lift/CL  ==
  CL0 : Inport
  CL_alpha : Inport  Port=2
  alpha : Inport  Port=3
  Add : Sum
  Product : Product
  "CL " : Outport
  wires:
  CL0/1 -> Add/1
  CL_alpha/1 -> Product/1
  Product/1 -> Add/2
  alpha/1 -> Product/2
  Add/1 -> "CL "/1

== system Despegue_model/Planta/Fuerzas y Momentos en Despegue/Transicion/Lift/Lift ==
  V : Inport
  S : Inport  Port=2
  rho : Inport  Port=3
  CL : Inport  Port=4
  "0.5 " : Constant  Value=0.5
  Product : Product  Inputs=6
  L : Outport
  wires:
  rho/1 -> Product/2
  V/1 -> Product/4, Product/5
  CL/1 -> Product/6
  Product/1 -> L/1
  S/1 -> Product/3
  "0.5 "/1 -> Product/1
